simulink model "Kalman_szuro"  (R2024a)
settings: Solver=ode1  StartTime=0.0  StopTime=8  FixedStep=0.033  RelTol=1e-3
values from neighbouring files (symbols this model uses):
  A = [0  1                           0                       0 ... (first row only)    [Inicializalas.m]
  Ad = get(sysd, 'A')    [Inicializalas.m]
  B1 = [0; 2*Cf/m; 0; 2*Cf*lf/Iz]    [Inicializalas.m]
  B1d = Bd(1:4,1)    [Inicializalas.m]
  B2 = [0; -(2*Cf*lf-2*Cr*lr)/(m*v)-v; 0; -(2*Cf*lf^2+2*Cr*lr^2)/(Iz*v)]    [Inicializalas.m]
  B2d = Bd(1:4,2)    [Inicializalas.m]
  C = [1 0 0 0 ... (first row only)    [Inicializalas.m]
  lf = 1236e-3    (= 1.236)    [Inicializalas.m]
  lr = 2789e-3 - lf    (= 1.553)    [Inicializalas.m]
  Qd = [Ts^3*Q1/3 Ts^2*Q1/2   0           0 ... (first row only)    [Inicializalas.m]
  R1 = 1e-2    (= 0.01)    [Inicializalas.m]
  R2 = deg2rad(1)^2    [Inicializalas.m]
  Rd = [R1 0 ... (first row only)    [Inicializalas.m]
  Ts = 0.033    [Inicializalas.m]
  v = 2    [Inicializalas.m]
undefined symbols (not defined in the file or in its folder): R
settings Model: Creator=PZs  LastModifiedBy=PZs
settings DataIOCC: SaveOutput=off  SignalLogging=off  DSMLogging=off  SaveTime=off  ReturnWorkspaceOutputs=off

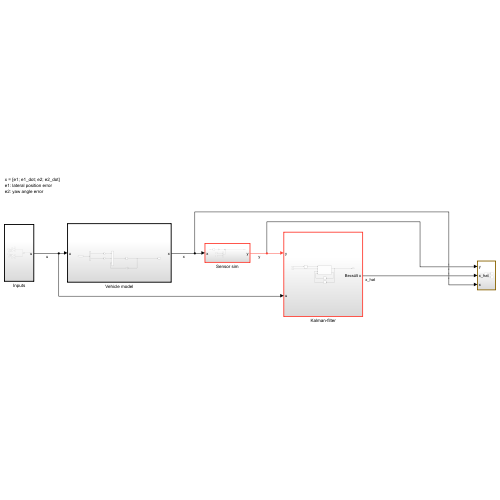
[thumbnail: Simulink's stored preview of the top-level diagram]
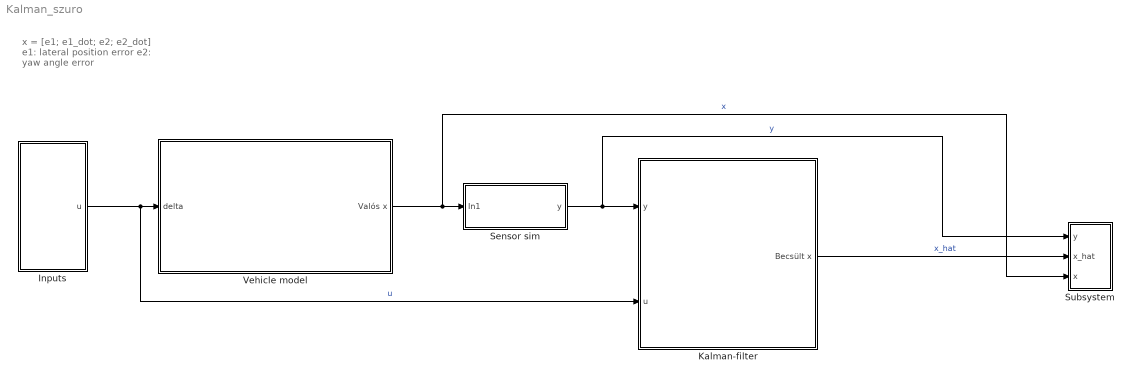
== system Kalman_szuro ==
  note: x = [e1; e1_dot; e2; e2_dot]
      | e1: lateral position error
      | e2: yaw angle error
  Inputs : Subsystem
  Kalman-filter : Subsystem
  Sensor sim : Subsystem
  Subsystem : Subsystem
  Vehicle model : Subsystem
  wires:
  Vehicle model/1(Valós x) -> Subsystem/3(x), Sensor sim/1(In1)  "x"
  Sensor sim/1(y) -> Subsystem/1(y), Kalman-filter/1(y)  "y"
  Inputs/1(u) -> Kalman-filter/2(u), Vehicle model/1(delta)  "u"
  Kalman-filter/1(Becsült x) -> Subsystem/2(x_hat)  "x_hat"

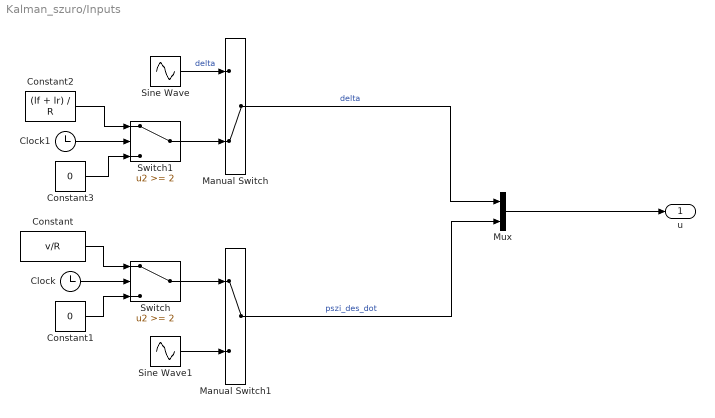
== system Kalman_szuro/Inputs ==
  Clock : Clock
  Clock1 : Clock
  Constant : Constant  Value=v/R
  Constant1 : Constant  Value=0
  Constant2 : Constant  Value=(lf + lr) / R
  Constant3 : Constant  Value=0
  Manual Switch : ManualSwitch  CurrentSetting=0
  Manual Switch1 : ManualSwitch
  Mux : Mux  Inputs=2
  Sine Wave : Sin  Amplitude=(lf + lr) / R  Frequency=2  SampleTime=0
  Sine Wave1 : Sin  Amplitude=v / R  Frequency=2  SampleTime=0
  Switch : Switch  Threshold=2  SaturateOnIntegerOverflow=off  InputSameDT=off
  Switch1 : Switch  Threshold=2  SaturateOnIntegerOverflow=off  InputSameDT=off
  u : Outport
  wires:
  Constant/1 -> Switch/1
  Manual Switch1/1 -> Mux/2  "pszi_des_dot"
  Clock/1 -> Switch/2
  Clock1/1 -> Switch1/2
  Constant3/1 -> Switch1/3
  Manual Switch/1 -> Mux/1  "delta"
  Constant1/1 -> Switch/3
  Mux/1 -> u/1
  Constant2/1 -> Switch1/1
  Switch1/1 -> Manual Switch/2
  Sine Wave/1 -> Manual Switch/1  "delta"
  Sine Wave1/1 -> Manual Switch1/2
  Switch/1 -> Manual Switch1/1

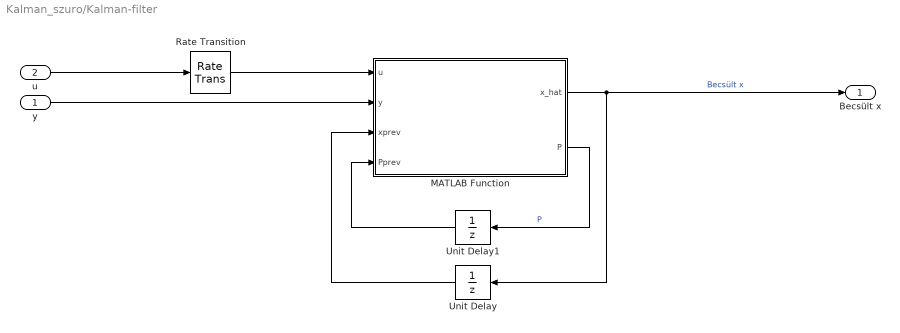
== system Kalman_szuro/Kalman-filter ==
  y : Inport
  u : Inport  Port=2
  MATLAB Function : MATLAB Function  TreatAsAtomicUnit=on
  Rate Transition : RateTransition  OutPortSampleTime=Ts
  Unit Delay : UnitDelay  InitialCondition=[0; 0; 0; 0]  SampleTime=-1  HasFrameUpgradeWarning=on
  Unit Delay1 : UnitDelay  InitialCondition=diag([10000, 10000, 10000, 10000])  SampleTime=-1  HasFrameUpgradeWarning=on
  Becsült x : Outport
  wires:
  Unit Delay1/1 -> MATLAB Function/4(Pprev)
  MATLAB Function/1(x_hat) -> Becsült x/1, Unit Delay/1  "Becsült x"
  MATLAB Function/2(P) -> Unit Delay1/1  "P"
  Unit Delay/1 -> MATLAB Function/3(xprev)
  u/1 -> Rate Transition/1
  y/1 -> MATLAB Function/2(y)
  Rate Transition/1 -> MATLAB Function/1(u)

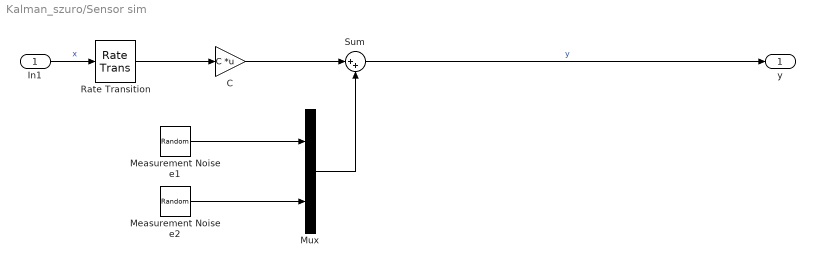
== system Kalman_szuro/Sensor sim ==
  In1 : Inport
  C : Gain  Gain=C  Multiplication=Matrix(K*u)
  Measurement Noise e1 : RandomNumber  Variance=R1  SampleTime=Ts
  Measurement Noise e2 : RandomNumber  Variance=R2  Seed=1  SampleTime=Ts
  Mux : Mux  Inputs=2
  Rate Transition : RateTransition  OutPortSampleTime=Ts
  Sum : Sum  Inputs=|++
  y : Outport
  wires:
  In1/1 -> Rate Transition/1  "x"
  Sum/1 -> y/1  "y"
  C/1 -> Sum/1
  Mux/1 -> Sum/2
  Rate Transition/1 -> C/1
  Measurement Noise e1/1 -> Mux/1
  Measurement Noise e2/1 -> Mux/2

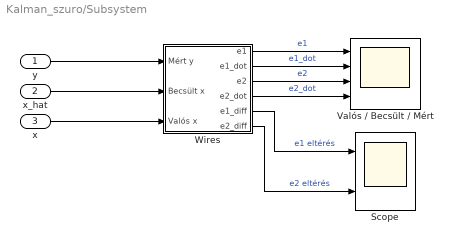
== system Kalman_szuro/Subsystem ==
  y : Inport
  x_hat : Inport  Port=2
  x : Inport  Port=3
  Scope : Scope  NumInputPorts=2
  Valós / Becsült / Mért : Scope  NumInputPorts=4
  Wires : Subsystem
  wires:
  Wires/3(e2) -> Valós / Becsült / Mért/3  "e2"
  Wires/2(e1_dot) -> Valós / Becsült / Mért/2  "e1_dot"
  Wires/4(e2_dot) -> Valós / Becsült / Mért/4  "e2_dot"
  Wires/6(e2_diff) -> Scope/2  "e2 eltérés"
  Wires/5(e1_diff) -> Scope/1  "e1 eltérés"
  Wires/1(e1) -> Valós / Becsült / Mért/1  "e1"
  x_hat/1 -> Wires/2(Becsült x)
  x/1 -> Wires/3(Valós x)
  y/1 -> Wires/1(Mért y)

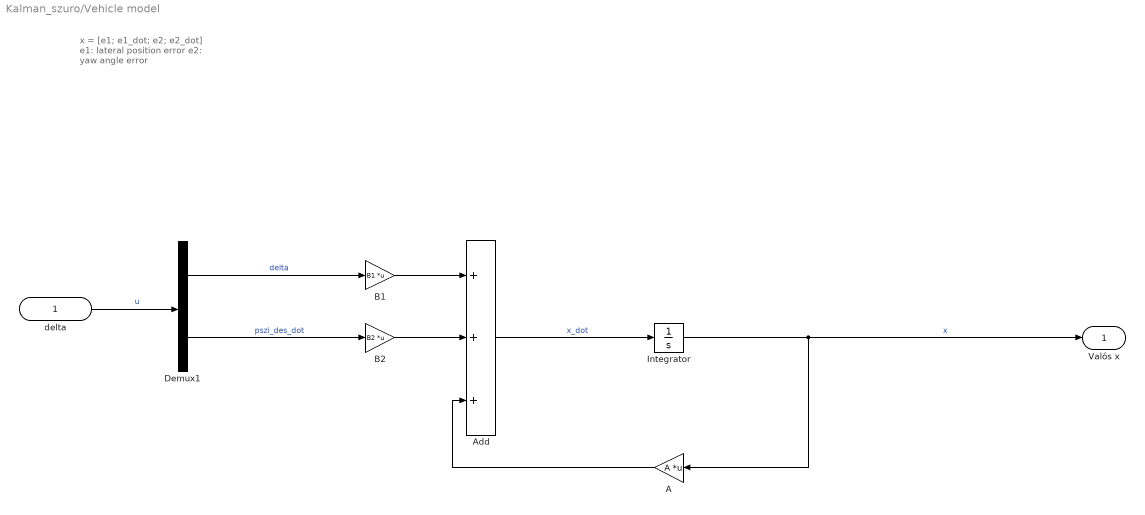
== system Kalman_szuro/Vehicle model ==
  note: x = [e1; e1_dot; e2; e2_dot]
      | e1: lateral position error
      | e2: yaw angle error
  delta : Inport
  A : Gain  Gain=A  Multiplication=Matrix(K*u)
  Add : Sum  Inputs=+++
  B1 : Gain  Gain=B1  Multiplication=Matrix(K*u)
  B2 : Gain  Gain=B2  Multiplication=Matrix(K*u)
  Demux1 : Demux  Outputs=2
  Integrator : Integrator
  Valós x : Outport
  wires:
  B2/1 -> Add/2
  Add/1 -> Integrator/1  "x_dot"
  Demux1/1 -> B1/1  "delta"
  B1/1 -> Add/1
  A/1 -> Add/3
  Demux1/2 -> B2/1  "pszi_des_dot"
  Integrator/1 -> Valós x/1, A/1  "x"
  delta/1 -> Demux1/1  "u"

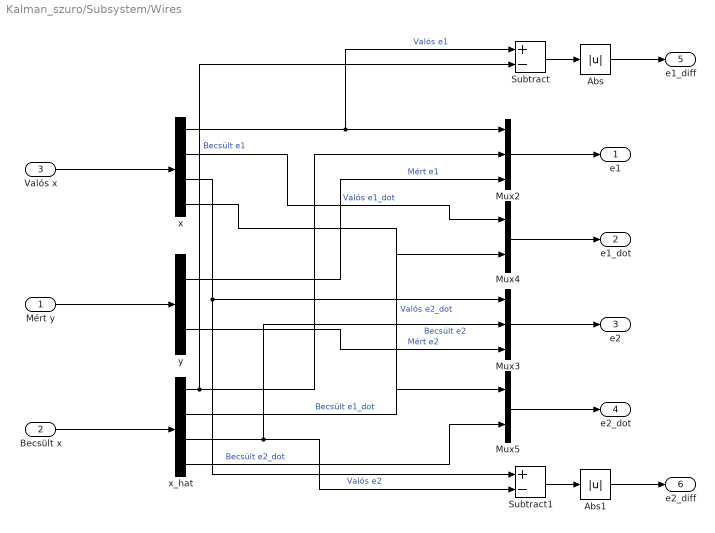
== system Kalman_szuro/Subsystem/Wires ==
  Mért y : Inport
  Becsült x : Inport  Port=2
  Valós x : Inport  Port=3
  Abs : Abs  SaturateOnIntegerOverflow=off
  Abs1 : Abs  SaturateOnIntegerOverflow=off
  Mux2 : Mux  Inputs=3
  Mux3 : Mux  Inputs=3
  Mux4 : Mux  Inputs=2
  Mux5 : Mux  Inputs=2
  Subtract : Sum  Inputs=+-
  Subtract1 : Sum  Inputs=+-
  x : Demux
  x_hat : Demux
  y : Demux  Outputs=2
  e1 : Outport
  e1_dot : Outport  Port=2
  e2 : Outport  Port=3
  e2_dot : Outport  Port=4
  e1_diff : Outport  Port=5
  e2_diff : Outport  Port=6
  wires:
  y/1 -> Mux2/3  "Mért e1"
  Mux4/1 -> e1_dot/1
  Valós x/1 -> x/1
  y/2 -> Mux3/3  "Mért e2"
  Mux3/1 -> e2/1
  x/2 -> Mux4/1  "Valós e1_dot"
  x_hat/4 -> Mux5/2  "Becsült e2_dot"
  x/3 -> Subtract1/1, Mux3/1  "Valós e2"
  Mux2/1 -> e1/1
  Mért y/1 -> y/1
  x/1 -> Subtract/1, Mux2/1  "Valós e1"
  x/4 -> Mux5/1  "Valós e2_dot"
  x_hat/3 -> Subtract1/2, Mux3/2  "Becsült e2"
  x_hat/2 -> Mux4/2  "Becsült e1_dot"
  x_hat/1 -> Subtract/2, Mux2/2  "Becsült e1"
  Mux5/1 -> e2_dot/1
  Becsült x/1 -> x_hat/1
  Subtract/1 -> Abs/1
  Subtract1/1 -> Abs1/1
  Abs1/1 -> e2_diff/1
  Abs/1 -> e1_diff/1

== matlab function Kalman_szuro/Kalman-filter/MATLAB Function ==
  data: u input; x_hat output; y input; xprev input; Pprev input; P output; Ad parameter; Qd parameter; Rd parameter; C parameter; B1d parameter; B2d parameter
function [x_hat, P] = Observer(u, y, xprev, Pprev, Ad, Qd, Rd, C, B1d, B2d)
   
    
    x_mid = Ad * xprev + B1d * u(1) + B2d * u(2);
    P_mid = Ad * Pprev * Ad' + Qd;

    K = P_mid * C' / (C * P_mid * C' + Rd);
    x_hat = x_mid + K * (y - C * x_mid);
    P = (eye(4) - K * C) * P_mid; 
    %x_hat(2) = 0;
end
